simulink model "ex1model"  (R2022b)
settings: Solver=VariableStepAuto  StartTime=0.0  StopTime=10.0  RelTol=1e-3
settings Model: Creator=Asus  LastModifiedBy=Asus

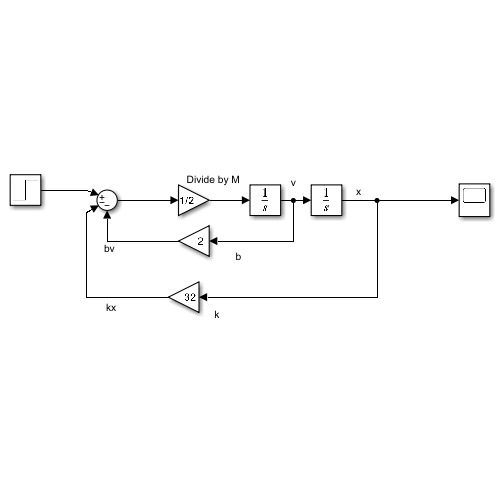
[thumbnail: Simulink's stored preview of the top-level diagram]
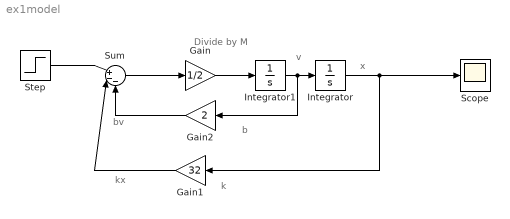
== system ex1model ==
  note: b
  note: k
  note: x
  note: bv
  note: kx
  note: v
  note: Divide by M
  Gain : Gain  Gain=1/2
  Gain1 : Gain  Gain=32
  Gain2 : Gain  Gain=2
  Integrator : Integrator
  Integrator1 : Integrator
  Scope : Scope
  Step : Step  SampleTime=0
  Sum : Sum  Inputs=|+--
  wires:
  Sum/1 -> Gain/1
  Step/1 -> Sum/1
  Gain1/1 -> Sum/2
  Gain/1 -> Integrator1/1
  Integrator/1 -> Gain1/1, Scope/1
  Integrator1/1 -> Gain2/1, Integrator/1
  Gain2/1 -> Sum/3
